simulink model "EcoSIM3_P2_C2_WIP"  (R2014b)
settings: Solver=ode1  SolverMode=SingleTasking  StartTime=0.0  StopTime=inf  FixedStep=0.01  RelTol=1e-3
PostLoadFcn:
  | %, if any(exist('dsrtsu_mdlpostloadfcn', 'file') == [2, 3, 6]), try dsrtsu_mdlpostloadfcn('Execute', bdroot); catch fprintf('Error in PostLoadFcn (dsrtsu_mdlpostloadfcn) for model "%s":\n %s\n', bdroot, lasterr); end, end,
InitFcn:
  | tic
  | %Startup_EcoSIM
values from neighbouring files (symbols this model uses):
  EngPwr = [0 5	10	15	20	25	30	35	40	45	50	55	60	65	70	75	80	85	90	95	100	105	110	115]    [Series_Maps.m]
  EngSpd = [0 477.4645 954.929 1909.858 2864.787 3819.716 4774.645 5729.574 6684.503]    [Series_Maps.m]
  EngTrq = [0	0	0	0	0	0	0	0	0	0	0	0	0	0	0	0	0	0	0	0	0	0	0	0 ... (first row only)    [Series_Maps.m]
  Power = [0 5 10 15 20 25 30]    [Series_Maps.m]
  Torque = [-50,-40,-30,-25,-20,-15,-10,-8,-6,-4,-2,0]    [Series_Maps.m]
undefined symbols (not defined in the file or in its folder): canChannel, Controls, DriveCycles, Driver, EM_EFF_MAP, EM_PwrLoss_MAP, Glbl, Overwritten_Mode, Plants, sigbuilder_block, Trialmap, Veh_Dynamics
libraries: simulink x141, canmsglib x113, fl_lib x104, canlib x89, nesl_utility x56, sdl_lib x29, dspsigops x6, dspswit3 x5, dspstat3 x2, commnoisgen2 x1, dspfdesign x1
(part 18 of 21)

== system EcoSIM3_P2_C2_WIP/Powertrain/Soft_ECUs_IO/VNT Vector/CANTx/ESS/BCM_Status ==
  ESS : Inport
  Bus Selector3 : BusSelector  OutputSignals=BCM_Status.bcm_chg_done,BCM_Status.bcm_chgc_stat,BCM_Status.bcm_cpwr_cmd,BCM_Status.bcm_cpwr_mon,BCM_Status.bcm_epo,BCM_Status.bcm_hvil_mon,BCM_Status.bcm_ibat,BCM_Status.bcm_mainc_stat,BCM_Status.bcm_on_plug,BCM_Status.bcm_ready,BCM_Status.bcm_soc,BCM_Status.bcm_vbat
  CAN Pack2 : canmsglib/CAN Pack  CANdbFile=C:\Users\EcoCAR_HIL\Documents\Khanna\EcoSIM3_P1_0_PHEV_TCU\Final_DBC\BCM_VehBus_Std.dbc  MsgList=BCM_Status  MsgName=BCM_Status  MsgIDType=Standard (11-bit identifier)  MsgIdentifier=1040  MsgLength=8  SignalInfo=bcm_alarm$14$2$2$2$1$0$1$0$0$3$#bcm_chg_done$52$1$2$2$1$0$1$0$0$1$#bcm_chgc_stat$6$2$2$2$1$0$1$0$0$2$#bcm_cool_req$53$1$2$2$1$0$1$0$0$1$#bcm_cpwr_cmd$12$1$2$2$1$0$1$0$0$1$#bcm_cpwr_mon$13$1$2$2$1$0$1$0$0$1$#bcm_epo$1$1$2$2$1$0$1$0$0$1$#bcm_gfd$16$12$2$2$1$0$2.500000e-01$0$0$1000$#bcm_hvil_mon$3$1$2$2$1$0$1$0$0$1$#bcm_ibat$40$16$2$2$1$0$2.500000e-02$-1000$-1000$500$#bcm_lls_status$54$2$2$2$1$0$1$0$0$3$#bcm_mainc_stat$4$2$2$2$1$0$1$0$0$2$#bcm_on_plug$2$1$2$2$1$0$1$0$0$1$#bcm_ready$0$1$2$2$1$0$1$0$0$1$#bcm_soc$24$8$2$2$1$0$5.000000e-01$0$0$100$#bcm_vbat$56$12$2$2$1$0$2.500000e-01$0$0$1000$#  NSignals=16  StartBits=str2num('[int32(14);int32(52);int32(6);int32(53);int32(12);int32(13);int32(1);int32(16);int32(3);int32(40);int32(54);int32(4);int32(2);int32(0);int32(24);int32(56)]')  SignalSizes=str2num('[int32(2);int32(1);int32(2);int32(1);int32(1);int32(1);int32(1);int32(12);int32(1);int32(16);int32(2);int32(2);int32(1);int32(1);int32(8);int32(12)]')  ByteOrders=str2num('[int32(2);int32(2);int32(2);int32(2);int32(2);int32(2);int32(2);int32(2);int32(2);int32(2);int32(2);int32(2);int32(2);int32(2);int32(2);int32(2)]')  DataTypes=str2num('[int32(2);int32(2);int32(2);int32(2);int32(2);int32(2);int32(2);int32(2);int32(2);int32(2);int32(2);int32(2);int32(2);int32(2);int32(2);int32(2)]')  MultiplexTypes=str2num('[int32(1);int32(1);int32(1);int32(1);int32(1);int32(1);int32(1);int32(1);int32(1);int32(1);int32(1);int32(1);int32(1);int32(1);int32(1);int32(1)]')  MultiplexValues=str2num('[double(0);double(0);double(0);double(0);double(0);double(0);double(0);double(0);double(0);double(0);double(0);double(0);double(0);double(0);double(0);double(0)]')  Factors=str2num('[double(1);double(1);double(1);double(1);double(1);double(1);double(1);double(2.500000e-01);double(1);double(2.500000e-02);double(1);double(1);double(1);double(1);double(5.000000e-01);double(2.500000e-01)]')  Offsets=str2num('[double(0);double(0);double(0);double(0);double(0);double(0);double(0);double(0);double(0);double(-1000);double(0);double(0);double(0);double(0);double(0);double(0)]')  Minimums=str2num('[double(0);double(0);double(0);double(0);double(0);double(0);double(0);double(0);double(0);double(-1000);double(0);double(0);double(0);double(0);double(0);double(0)]')  Maximums=str2num('[double(3);double(1);double(2);double(1);double(1);double(1);double(1);double(1000);double(1);double(500);double(3);double(2);double(1);double(1);double(100);double(1000)]')  Remote=off
      settings: DataFormat=CANdb specified signals
  CAN Transmit6 : canlib/CAN Transmit  BlockHandle=7345.0001  DeviceMenu=(none)  Device=Vector Virtual 1 (Channel 1)  ObjConstructor=canChannel('Vector', 'Virtual 1', 1)  EnablePeriodicTransmit=off  MessagePeriod=1.000
  Ground{2..5} (4 alike) : Ground
  Rate Transition : RateTransition
  Rate Transition1 : RateTransition
  Rate Transition10 : RateTransition  Deterministic=off
  Rate Transition11 : RateTransition  Deterministic=off
  Rate Transition9 : RateTransition  Deterministic=off
  wires:
  Rate Transition10/1 -> CAN Pack2/10
  Rate Transition9/1 -> CAN Pack2/16
  Rate Transition11/1 -> CAN Pack2/15
  Ground3/1 -> CAN Pack2/8
  Ground2/1 -> CAN Pack2/4
  Ground5/1 -> CAN Pack2/11
  Bus Selector3/3 -> CAN Pack2/5  "<bcm_cpwr_cmd>"
  Bus Selector3/4 -> CAN Pack2/6  "<bcm_cpwr_mon>"
  Bus Selector3/2 -> Rate Transition/1  "<bcm_chgc_stat>"
  ESS/1 -> Bus Selector3/1
  Bus Selector3/5 -> CAN Pack2/7  "<bcm_epo>"
  Bus Selector3/6 -> CAN Pack2/9  "<bcm_hvil_mon>"
  Bus Selector3/8 -> CAN Pack2/12  "<bcm_mainc_stat>"
  Bus Selector3/7 -> Rate Transition10/1  "<bcm_ibat>"
  Bus Selector3/9 -> CAN Pack2/13  "<bcm_on_plug>"
  Bus Selector3/10 -> CAN Pack2/14  "<bcm_ready>"
  Bus Selector3/11 -> Rate Transition11/1  "<bcm_soc>"
  Bus Selector3/12 -> Rate Transition9/1  "<bcm_vbat>"
  Rate Transition/1 -> CAN Pack2/3
  CAN Pack2/1 -> CAN Transmit6/1
  Ground4/1 -> CAN Pack2/1
  Bus Selector3/1 -> Rate Transition1/1  "<bcm_chg_done>"
  Rate Transition1/1 -> CAN Pack2/2

== system EcoSIM3_P2_C2_WIP/Powertrain/Soft_ECUs_IO/VNT Vector/CANTx/GMLAN/PPEI_Brake_Apply_Status ==
  GM : Inport
  Bus Selector3 : BusSelector  OutputSignals=PPEI_Brake_Apply_Status.BrkPdlPos
  CAN Pack1 : canmsglib/CAN Pack  CANdbFile=C:\Users\EcoCAR_HIL\Documents\Khanna\EcoSIM3_P1_0_PHEV_TCU\Final_DBC\GlobalAHS_anon GM CONFIDENTIAL.dbc  MsgList=PPEI_Brake_Apply_Status  MsgName=PPEI_Brake_Apply_Status  MsgIDType=Standard (11-bit identifier)  MsgIdentifier=241  MsgLength=6  SignalInfo=BrkAppSnsrHmPosLrnd$30$1$2$2$1$0$1$0$0$1$#BrkPdlChkData$40$17$2$2$1$0$1$0$0$131071$#BrkPdlInTrvPrt$2$2$2$2$1$0$1$0$0$3$#BrkPdlModTrvl$6$1$2$2$1$0$1$0$0$1$#BrkPdlModTrvlV$7$1$2$2$1$0$1$0$0$1$#BrkPdlPos$8$8$2$2$1$0$3.921570e-01$0$0$1.000000e+02$#BrkPdlPosGrad$16$8$2$1$1$0$40$0$-5120$5080$#BrkPedPosAlvRolngCnt$4$2$2$2$1$0$1$0$0$3$#BrkPedTrvlAchvd$1$1$2$2$1$0$1$0$0$1$#BrkPedTrvlAchvdV$0$1$2$2$1$0$1$0$0$1$#NotEventStat$28$2$2$2$1$0$1$0$0$3$#  NSignals=11  StartBits=str2num('[int32(30);int32(40);int32(2);int32(6);int32(7);int32(8);int32(16);int32(4);int32(1);int32(0);int32(28)]')  SignalSizes=str2num('[int32(1);int32(17);int32(2);int32(1);int32(1);int32(8);int32(8);int32(2);int32(1);int32(1);int32(2)]')  ByteOrders=str2num('[int32(2);int32(2);int32(2);int32(2);int32(2);int32(2);int32(2);int32(2);int32(2);int32(2);int32(2)]')  DataTypes=str2num('[int32(2);int32(2);int32(2);int32(2);int32(2);int32(2);int32(1);int32(2);int32(2);int32(2);int32(2)]')  MultiplexTypes=str2num('[int32(1);int32(1);int32(1);int32(1);int32(1);int32(1);int32(1);int32(1);int32(1);int32(1);int32(1)]')  MultiplexValues=str2num('[double(0);double(0);double(0);double(0);double(0);double(0);double(0);double(0);double(0);double(0);double(0)]')  Factors=str2num('[double(1);double(1);double(1);double(1);double(1);double(3.921570e-01);double(40);double(1);double(1);double(1);double(1)]')  Offsets=str2num('[double(0);double(0);double(0);double(0);double(0);double(0);double(0);double(0);double(0);double(0);double(0)]')  Minimums=str2num('[double(0);double(0);double(0);double(0);double(0);double(0);double(-5120);double(0);double(0);double(0);double(0)]')  Maximums=str2num('[double(1);double(131071);double(3);double(1);double(1);double(1.000000e+02);double(5080);double(3);double(1);double(1);double(3)]')  Remote=off
      settings: DataFormat=CANdb specified signals
  Ground_{1..10} (10 alike) : Ground
  Rate Transition : RateTransition
  Out1 : Outport
  wires:
  Ground_1/1 -> CAN Pack1/1
  Ground_5/1 -> CAN Pack1/5
  Ground_4/1 -> CAN Pack1/4
  Ground_6/1 -> CAN Pack1/7
  Ground_2/1 -> CAN Pack1/2
  Ground_3/1 -> CAN Pack1/3
  Ground_10/1 -> CAN Pack1/11
  Ground_7/1 -> CAN Pack1/8
  Ground_8/1 -> CAN Pack1/9
  Ground_9/1 -> CAN Pack1/10
  Bus Selector3/1 -> Rate Transition/1  "<BrkPdlPos>"
  GM/1 -> Bus Selector3/1
  Rate Transition/1 -> CAN Pack1/6
  CAN Pack1/1 -> Out1/1

== system EcoSIM3_P2_C2_WIP/Powertrain/Soft_ECUs_IO/VNT Vector/CANTx/GMLAN/PPEI_Driven_Whl_Rotational_Stat ==
  GM : Inport
  Bus Selector2 : BusSelector  OutputSignals=PPEI_Driven_Whl_Rotational_Stat.WRSLDWhlDistPlsCntr,PPEI_Driven_Whl_Rotational_Stat.WRSRDWhlDistPlsCntr
  CAN Pack4 : canmsglib/CAN Pack  CANdbFile=C:\Users\EcoCAR_HIL\Documents\Khanna\EcoSIM3_P1_0_PHEV_TCU\Final_DBC\GlobalAHS_anon GM CONFIDENTIAL.dbc  MsgList=PPEI_Driven_Whl_Rotational_Stat  MsgName=PPEI_Driven_Whl_Rotational_Stat  MsgIDType=Standard (11-bit identifier)  MsgIdentifier=193  MsgLength=8  SignalInfo=WRSLDSeqNum$4$2$2$2$1$0$1$0$0$3$#WRSLDWhlDisTpRC$6$2$2$2$1$0$1$0$0$3$#WRSLDWhlDistPlsCntr$8$10$2$2$1$0$1$0$0$1023$#WRSLDWhlDistTmstm$24$16$2$2$1$0$1$0$0$65535$#WRSLDWhlDistVal$2$1$2$2$1$0$1$0$0$1$#WRSLDWhlRotStatRst$3$1$2$2$1$0$1$0$0$1$#WRSRDSeqNum$36$2$2$2$1$0$1$0$0$3$#WRSRDWhlDisTpRC$38$2$2$2$1$0$1$0$0$3$#WRSRDWhlDistPlsCntr$40$10$2$2$1$0$1$0$0$1023$#WRSRDWhlDistTmstm$56$16$2$2$1$0$1$0$0$65535$#WRSRDWhlDistVal$34$1$2$2$1$0$1$0$0$1$#WRSRDWhlRotStatRst$35$1$2$2$1$0$1$0$0$1$#  NSignals=12  StartBits=str2num('[int32(4);int32(6);int32(8);int32(24);int32(2);int32(3);int32(36);int32(38);int32(40);int32(56);int32(34);int32(35)]')  SignalSizes=str2num('[int32(2);int32(2);int32(10);int32(16);int32(1);int32(1);int32(2);int32(2);int32(10);int32(16);int32(1);int32(1)]')  ByteOrders=str2num('[int32(2);int32(2);int32(2);int32(2);int32(2);int32(2);int32(2);int32(2);int32(2);int32(2);int32(2);int32(2)]')  DataTypes=str2num('[int32(2);int32(2);int32(2);int32(2);int32(2);int32(2);int32(2);int32(2);int32(2);int32(2);int32(2);int32(2)]')  MultiplexTypes=str2num('[int32(1);int32(1);int32(1);int32(1);int32(1);int32(1);int32(1);int32(1);int32(1);int32(1);int32(1);int32(1)]')  MultiplexValues=str2num('[double(0);double(0);double(0);double(0);double(0);double(0);double(0);double(0);double(0);double(0);double(0);double(0)]')  Factors=str2num('[double(1);double(1);double(1);double(1);double(1);double(1);double(1);double(1);double(1);double(1);double(1);double(1)]')  Offsets=str2num('[double(0);double(0);double(0);double(0);double(0);double(0);double(0);double(0);double(0);double(0);double(0);double(0)]')  Minimums=str2num('[double(0);double(0);double(0);double(0);double(0);double(0);double(0);double(0);double(0);double(0);double(0);double(0)]')  Maximums=str2num('[double(3);double(3);double(1023);double(65535);double(1);double(1);double(3);double(3);double(1023);double(65535);double(1);double(1)]')  Remote=off
      settings: DataFormat=CANdb specified signals
  CAN Transmit : canlib/CAN Transmit  BlockHandle=7430.0001  DeviceMenu=(none)  Device=Vector Virtual 1 (Channel 1)  ObjConstructor=canChannel('Vector', 'Virtual 1', 1)  EnablePeriodicTransmit=on  MessagePeriod=0.01
  Ground_{50..59} (10 alike) : Ground
  Scope1 : Scope
      settings: SaveName=ScopeData18
  Scope2 : Scope
      settings: SaveName=ScopeData23
  Out1 : Outport
  wires:
  Bus Selector2/1 -> Scope2/1, CAN Pack4/3, Scope1/1  "<WRSLDWhlDistPlsCntr>"
  Bus Selector2/2 -> CAN Pack4/9  "<WRSRDWhlDistPlsCntr>"
  Ground_57/1 -> CAN Pack4/10
  Ground_50/1 -> CAN Pack4/1
  Ground_59/1 -> CAN Pack4/12
  Ground_53/1 -> CAN Pack4/5
  Ground_52/1 -> CAN Pack4/4
  Ground_51/1 -> CAN Pack4/2
  Ground_54/1 -> CAN Pack4/6
  Ground_55/1 -> CAN Pack4/7
  Ground_56/1 -> CAN Pack4/8
  Ground_58/1 -> CAN Pack4/11
  GM/1 -> Bus Selector2/1
  CAN Pack4/1 -> CAN Transmit/1, Out1/1

== system EcoSIM3_P2_C2_WIP/Powertrain/Soft_ECUs_IO/VNT Vector/CANTx/GMLAN/PPEI_NonDrivn_Whl_Rotational_Stat ==
  GM : Inport
  Bus Selector5 : BusSelector  OutputSignals=PPEI_NonDrivn_Whl_Rotationl_Stat.WRSLNDWhlDistPCntr,PPEI_NonDrivn_Whl_Rotationl_Stat.WRSRNDWhlDistPCntr
  CAN Pack5 : canmsglib/CAN Pack  CANdbFile=C:\Users\EcoCAR_HIL\Documents\Khanna\EcoSIM3_P1_0_PHEV_TCU\Final_DBC\GlobalAHS_anon GM CONFIDENTIAL.dbc  MsgList=PPEI_NonDrivn_Whl_Rotationl_Stat  MsgName=PPEI_NonDrivn_Whl_Rotationl_Stat  MsgIDType=Standard (11-bit identifier)  MsgIdentifier=197  MsgLength=8  SignalInfo=WRSLNDSeqNum$4$2$2$2$1$0$1$0$0$3$#WRSLNDWhlDisTpRC$6$2$2$2$1$0$1$0$0$3$#WRSLNDWhlDistPCntr$8$10$2$2$1$0$1$0$0$1023$#WRSLNDWhlDistTstm$24$16$2$2$1$0$1$0$0$65535$#WRSLNDWhlDistVal$2$1$2$2$1$0$1$0$0$1$#WRSLNDWhlRotStRst$3$1$2$2$1$0$1$0$0$1$#WRSRNDSeqNum$36$2$2$2$1$0$1$0$0$3$#WRSRNDWhlDisTpRC$38$2$2$2$1$0$1$0$0$3$#WRSRNDWhlDistPCntr$40$10$2$2$1$0$1$0$0$1023$#WRSRNDWhlDistTstm$56$16$2$2$1$0$1$0$0$65535$#WRSRNDWhlDistVal$34$1$2$2$1$0$1$0$0$1$#WRSRNDWhlRotStRst$35$1$2$2$1$0$1$0$0$1$#  NSignals=12  StartBits=str2num('[int32(4);int32(6);int32(8);int32(24);int32(2);int32(3);int32(36);int32(38);int32(40);int32(56);int32(34);int32(35)]')  SignalSizes=str2num('[int32(2);int32(2);int32(10);int32(16);int32(1);int32(1);int32(2);int32(2);int32(10);int32(16);int32(1);int32(1)]')  ByteOrders=str2num('[int32(2);int32(2);int32(2);int32(2);int32(2);int32(2);int32(2);int32(2);int32(2);int32(2);int32(2);int32(2)]')  DataTypes=str2num('[int32(2);int32(2);int32(2);int32(2);int32(2);int32(2);int32(2);int32(2);int32(2);int32(2);int32(2);int32(2)]')  MultiplexTypes=str2num('[int32(1);int32(1);int32(1);int32(1);int32(1);int32(1);int32(1);int32(1);int32(1);int32(1);int32(1);int32(1)]')  MultiplexValues=str2num('[double(0);double(0);double(0);double(0);double(0);double(0);double(0);double(0);double(0);double(0);double(0);double(0)]')  Factors=str2num('[double(1);double(1);double(1);double(1);double(1);double(1);double(1);double(1);double(1);double(1);double(1);double(1)]')  Offsets=str2num('[double(0);double(0);double(0);double(0);double(0);double(0);double(0);double(0);double(0);double(0);double(0);double(0)]')  Minimums=str2num('[double(0);double(0);double(0);double(0);double(0);double(0);double(0);double(0);double(0);double(0);double(0);double(0)]')  Maximums=str2num('[double(3);double(3);double(1023);double(65535);double(1);double(1);double(3);double(3);double(1023);double(65535);double(1);double(1)]')  Remote=off
      settings: DataFormat=CANdb specified signals
  CAN Transmit : canlib/CAN Transmit  BlockHandle=7468.0001  DeviceMenu=(none)  Device=Vector Virtual 1 (Channel 1)  ObjConstructor=canChannel('Vector', 'Virtual 1', 1)  EnablePeriodicTransmit=on  MessagePeriod=0.01
  Ground_{60..69} (10 alike) : Ground
  Out1 : Outport
  wires:
  Bus Selector5/2 -> CAN Pack5/9  "<WRSRNDWhlDistPCntr>"
  Bus Selector5/1 -> CAN Pack5/3  "<WRSLNDWhlDistPCntr>"
  Ground_60/1 -> CAN Pack5/1
  Ground_69/1 -> CAN Pack5/12
  Ground_63/1 -> CAN Pack5/5
  Ground_61/1 -> CAN Pack5/2
  Ground_66/1 -> CAN Pack5/8
  Ground_67/1 -> CAN Pack5/10
  Ground_68/1 -> CAN Pack5/11
  Ground_65/1 -> CAN Pack5/7
  Ground_62/1 -> CAN Pack5/4
  GM/1 -> Bus Selector5/1
  CAN Pack5/1 -> CAN Transmit/1, Out1/1
  Ground_64/1 -> CAN Pack5/6

== system EcoSIM3_P2_C2_WIP/Powertrain/Soft_ECUs_IO/VNT Vector/CANTx/GMLAN/PPEI_Platform_General_Status ==
  GM : Inport
  Bus Selector1 : BusSelector  OutputSignals=PPEI_Platform_General_Status.SysPwrMd
  CAN Pack2 : canmsglib/CAN Pack  CANdbFile=C:\Users\EcoCAR_HIL\Documents\Khanna\EcoSIM3_P1_0_PHEV_TCU\Final_DBC\GlobalAHS_anon GM CONFIDENTIAL.dbc  MsgList=PPEI_Platform_General_Status  MsgName=PPEI_Platform_General_Status  MsgIDType=Standard (11-bit identifier)  MsgIdentifier=497  MsgLength=8  SignalInfo=ACCmpsrFldOn$63$1$2$2$1$0$1$0$0$1$#ACCompModReq$11$2$2$2$1$0$1$0$0$3$#ACCompNormLd$48$8$2$2$1$0$1.000000e-01$0$0$2.550000e+01$#ACCompNormLdV$10$1$2$2$1$0$1$0$0$1$#ACCompSysVDA$9$1$2$2$1$0$1$0$0$1$#ACCompSysVDM$60$1$2$2$1$0$1$0$0$1$#AirbgVDA$57$1$2$2$1$0$1$0$0$1$#BkupPwrModeMstrVDA$7$1$2$2$1$0$1$0$0$1$#BkupPwrModeMstrVDM$61$1$2$2$1$0$1$0$0$1$#DispMeasSys$59$1$2$2$1$0$1$0$0$1$#ElvtdIdlCstStReq$32$2$2$2$1$0$1$0$0$3$#EngOilLfRstRq$37$1$2$2$1$0$1$0$0$1$#FuelFltLfRstRqd$56$1$2$2$1$0$1$0$0$1$#ImmblzrPreRelPswdStat$8$1$2$2$1$0$1$0$0$1$#ImmblzrPreRelPswrd$24$16$2$2$1$0$1$0$0$65535$#PMMAccTrmSt$2$1$2$2$1$0$1$0$0$1$#PMMRunCrkTrmSt$3$1$2$2$1$0$1$0$0$1$#PTORSMstrEngShtReq$13$1$2$2$1$0$1$0$0$1$#PTORmStMsEngStRq$14$1$2$2$1$0$1$0$0$1$#PrkBrkSwAtv$36$1$2$2$1$0$1$0$0$1$#PrkBrkVDA$35$1$2$2$1$0$1$0$0$1$#PrkBrkVDM$62$1$2$2$1$0$1$0$0$1$#RmVehStrRq$15$1$2$2$1$0$1$0$0$1$#SIRDpl$58$1$2$2$1$0$1$0$0$1$#SysBkUpPwrMd$4$2$2$2$1$0$1$0$0$3$#SysBkupPwrMdEn$6$1$2$2$1$0$1$0$0$1$#SysPwrMd$0$2$2$2$1$0$1$0$0$3$#ThrtlPrgrsnReq$38$2$2$2$1$0$1$0$0$3$#TrStLgMdAtv$34$1$2$2$1$0$1$0$0$1$#  NSignals=29  StartBits=str2num('[int32(63);int32(11);int32(48);int32(10);int32(9);int32(60);int32(57);int32(7);int32(61);int32(59);int32(32);int32(37);int32(56);int32(8);int32(24);int32(2);int32(3);int32(13);int32(14);int32(36);int32(35);int32(62);int32(15);int32(58);int32(4);int32(6);int32(0);int32(38);int32(34)]')  SignalSizes=str2num('[int32(1);int32(2);int32(8);int32(1);int32(1);int32(1);int32(1);int32(1);int32(1);int32(1);int32(2);int32(1);int32(1);int32(1);int32(16);int32(1);int32(1);int32(1);int32(1);int32(1);int32(1);int32(1);int32(1);int32(1);int32(2);int32(1);int32(2);int32(2);int32(1)]')  ByteOrders=str2num('[int32(2);int32(2);int32(2);int32(2);int32(2);int32(2);int32(2);int32(2);int32(2);int32(2);int32(2);int32(2);int32(2);int32(2);int32(2);int32(2);int32(2);int32(2);int32(2);int32(2);int32(2);int32(2);int32(2);int32(2);int32(2);int32(2);int32(2);int32(2);int32(2)]')  DataTypes=str2num('[int32(2);int32(2);int32(2);int32(2);int32(2);int32(2);int32(2);int32(2);int32(2);int32(2);int32(2);int32(2);int32(2);int32(2);int32(2);int32(2);int32(2);int32(2);int32(2);int32(2);int32(2);int32(2);int32(2);int32(2);int32(2);int32(2);int32(2);int32(2);int32(2)]')  MultiplexTypes=str2num('[int32(1);int32(1);int32(1);int32(1);int32(1);int32(1);int32(1);int32(1);int32(1);int32(1);int32(1);int32(1);int32(1);int32(1);int32(1);int32(1);int32(1);int32(1);int32(1);int32(1);int32(1);int32(1);int32(1);int32(1);int32(1);int32(1);int32(1);int32(1);int32(1)]')  MultiplexValues=str2num('[double(0);double(0);double(0);double(0);double(0);double(0);double(0);double(0);double(0);double(0);double(0);double(0);double(0);double(0);double(0);double(0);double(0);double(0);double(0);double(0);double(0);double(0);double(0);double(0);double(0);double(0);double(0);double(0);double(0)]')  Factors=str2num('[double(1);double(1);double(1.000000e-01);double(1);double(1);double(1);double(1);double(1);double(1);double(1);double(1);double(1);double(1);double(1);double(1);double(1);double(1);double(1);double(1);double(1);double(1);double(1);double(1);double(1);double(1);double(1);double(1);double(1);double(1)]')  Offsets=str2num('[double(0);double(0);double(0);double(0);double(0);double(0);double(0);double(0);double(0);double(0);double(0);double(0);double(0);double(0);double(0);double(0);double(0);double(0);double(0);double(0);double(0);double(0);double(0);double(0);double(0);double(0);double(0);double(0);double(0)]')  Minimums=str2num('[double(0);double(0);double(0);double(0);double(0);double(0);double(0);double(0);double(0);double(0);double(0);double(0);double(0);double(0);double(0);double(0);double(0);double(0);double(0);double(0);double(0);double(0);double(0);double(0);double(0);double(0);double(0);double(0);double(0)]')  Maximums=str2num('[double(1);double(3);double(2.550000e+01);double(1);double(1);double(1);double(1);double(1);double(1);double(1);double(3);double(1);double(1);double(1);double(65535);double(1);double(1);double(1);double(1);double(1);double(1);double(1);double(1);double(1);double(3);double(1);double(3);double(3);double(1)]')  Remote=off
      settings: DataFormat=CANdb specified signals
  Ground_{11..38} (28 alike) : Ground
  Rate Transition : RateTransition
  Out1 : Outport
  wires:
  Ground_29/1 -> CAN Pack2/19
  CAN Pack2/1 -> Out1/1
  Ground_32/1 -> CAN Pack2/22
  Ground_35/1 -> CAN Pack2/25
  Ground_11/1 -> CAN Pack2/1
  Ground_27/1 -> CAN Pack2/17
  Ground_15/1 -> CAN Pack2/5
  Ground_37/1 -> CAN Pack2/28
  Ground_13/1 -> CAN Pack2/3
  Ground_16/1 -> CAN Pack2/6
  Ground_24/1 -> CAN Pack2/14
  Ground_25/1 -> CAN Pack2/15
  Ground_14/1 -> CAN Pack2/4
  Ground_28/1 -> CAN Pack2/18
  Ground_31/1 -> CAN Pack2/21
  Ground_38/1 -> CAN Pack2/29
  Ground_21/1 -> CAN Pack2/11
  Ground_26/1 -> CAN Pack2/16
  Ground_30/1 -> CAN Pack2/20
  Ground_20/1 -> CAN Pack2/10
  Ground_17/1 -> CAN Pack2/7
  Ground_22/1 -> CAN Pack2/12
  Ground_36/1 -> CAN Pack2/26
  Ground_33/1 -> CAN Pack2/23
  Ground_18/1 -> CAN Pack2/8
  Ground_34/1 -> CAN Pack2/24
  Ground_12/1 -> CAN Pack2/2
  Ground_19/1 -> CAN Pack2/9
  Ground_23/1 -> CAN Pack2/13
  Bus Selector1/1 -> Rate Transition/1  "<SysPwrMd>"
  GM/1 -> Bus Selector1/1
  Rate Transition/1 -> CAN Pack2/27

== system EcoSIM3_P2_C2_WIP/Powertrain/Soft_ECUs_IO/VNT Vector/CANTx/GMLAN/PPEI_Vehicle_Speed_and_Distance ==
  GM : Inport
  Bus Selector4 : BusSelector  OutputSignals=PPEI_Vehicle_Speed_and_Distance.VehSpdAvgDrvn
  CAN Pack3 : canmsglib/CAN Pack  CANdbFile=C:\Users\EcoCAR_HIL\Documents\Khanna\EcoSIM3_P1_0_PHEV_TCU\Final_DBC\GlobalAHS_anon GM CONFIDENTIAL.dbc  MsgList=PPEI_Vehicle_Speed_and_Distance  MsgName=PPEI_Vehicle_Speed_and_Distance  MsgIDType=Standard (11-bit identifier)  MsgIdentifier=1001  MsgLength=8  SignalInfo=DistRollCntAvgDrvn$24$13$2$2$1$0$1.250000e-01$0$0$1.023875e+03$#DistRollCntAvgDrvnSrc$55$1$2$2$1$0$1$0$0$1$#DistRollCntAvgDrvnV$22$1$2$2$1$0$1$0$0$1$#DstRolCntAvNDrRstOc$53$1$2$2$1$0$1$0$0$1$#DstRolCntAvgDrnRstOc$21$1$2$2$1$0$1$0$0$1$#DstRolCntAvgNonDrvn$56$13$2$2$1$0$1.250000e-01$0$0$1.023875e+03$#DstRolCntAvgNonDrvnV$54$1$2$2$1$0$1$0$0$1$#VehSpdAvgDrvn$8$15$2$2$1$0$1.562500e-02$0$0$5.119844e+02$#VehSpdAvgDrvnSrc$23$1$2$2$1$0$1$0$0$1$#VehSpdAvgDrvnV$7$1$2$2$1$0$1$0$0$1$#VehSpdAvgNDrvn$40$15$2$2$1$0$1.562500e-02$0$0$5.119844e+02$#VehSpdAvgNDrvnV$39$1$2$2$1$0$1$0$0$1$#  NSignals=12  StartBits=str2num('[int32(24);int32(55);int32(22);int32(53);int32(21);int32(56);int32(54);int32(8);int32(23);int32(7);int32(40);int32(39)]')  SignalSizes=str2num('[int32(13);int32(1);int32(1);int32(1);int32(1);int32(13);int32(1);int32(15);int32(1);int32(1);int32(15);int32(1)]')  ByteOrders=str2num('[int32(2);int32(2);int32(2);int32(2);int32(2);int32(2);int32(2);int32(2);int32(2);int32(2);int32(2);int32(2)]')  DataTypes=str2num('[int32(2);int32(2);int32(2);int32(2);int32(2);int32(2);int32(2);int32(2);int32(2);int32(2);int32(2);int32(2)]')  MultiplexTypes=str2num('[int32(1);int32(1);int32(1);int32(1);int32(1);int32(1);int32(1);int32(1);int32(1);int32(1);int32(1);int32(1)]')  MultiplexValues=str2num('[double(0);double(0);double(0);double(0);double(0);double(0);double(0);double(0);double(0);double(0);double(0);double(0)]')  Factors=str2num('[double(1.250000e-01);double(1);double(1);double(1);double(1);double(1.250000e-01);double(1);double(1.562500e-02);double(1);double(1);double(1.562500e-02);double(1)]')  Offsets=str2num('[double(0);double(0);double(0);double(0);double(0);double(0);double(0);double(0);double(0);double(0);double(0);double(0)]')  Minimums=str2num('[double(0);double(0);double(0);double(0);double(0);double(0);double(0);double(0);double(0);double(0);double(0);double(0)]')  Maximums=str2num('[double(1.023875e+03);double(1);double(1);double(1);double(1);double(1.023875e+03);double(1);double(5.119844e+02);double(1);double(1);double(5.119844e+02);double(1)]')  Remote=off
      settings: DataFormat=CANdb specified signals
  Ground_{39..49} (11 alike) : Ground
  Rate Transition : RateTransition
  Out1 : Outport
  wires:
  CAN Pack3/1 -> Out1/1
  Ground_47/1 -> CAN Pack3/10
  Ground_45/1 -> CAN Pack3/7
  Ground_44/1 -> CAN Pack3/6
  Ground_46/1 -> CAN Pack3/9
  Ground_49/1 -> CAN Pack3/12
  Ground_48/1 -> CAN Pack3/11
  Ground_42/1 -> CAN Pack3/4
  Ground_40/1 -> CAN Pack3/2
  Ground_39/1 -> CAN Pack3/1
  Ground_43/1 -> CAN Pack3/5
  Ground_41/1 -> CAN Pack3/3
  Bus Selector4/1 -> Rate Transition/1  "<VehSpdAvgDrvn>"
  GM/1 -> Bus Selector4/1
  Rate Transition/1 -> CAN Pack3/8

== system EcoSIM3_P2_C2_WIP/Supervisory Controller/Functional Safety1/Functional Safety Algorithm/Fault Detection (Team Developed)/Torque Security Faults/Torque Comparisons ==
  Torque Estimates : Inport
  Torque Feedbacks : Inport  Port=2
  Torque Requests : Inport  Port=3
  BAS Torque Comparison : Subsystem  Commented=on
  Belt Coupler Torque Comparison : Subsystem  Commented=on
  Bus Creator : BusCreator  Inputs=3
  Bus Creator1 : BusCreator  Inputs=9
  Clutch Torque Comparison : Subsystem  Commented=on
  Electric Motor Torque Comparison : Subsystem
  Engine Torque Comparison : Subsystem  Commented=on
  PTU Torque Comparison : Subsystem  Commented=on
  Rear Diff Torque Comparison : Subsystem  Commented=on
  Trans Torque Comparison : Subsystem  Commented=on
  Wheel Torque Comparison : Subsystem  Commented=on
  Faults : Outport
  wires:
  Bus Creator1/1 -> Faults/1  "Trq_Security_Faults"
  Torque Requests/1 -> Bus Creator/3
  Torque Feedbacks/1 -> Bus Creator/2
  Torque Estimates/1 -> Bus Creator/1
  Clutch Torque Comparison/1(Out1) -> Bus Creator1/9
  Rear Diff Torque Comparison/1(Out1) -> Bus Creator1/8
  PTU Torque Comparison/1(Out1) -> Bus Creator1/7
  Belt Coupler Torque Comparison/1(Out1) -> Bus Creator1/6
  Trans Torque Comparison/1(Out1) -> Bus Creator1/5
  Electric Motor Torque Comparison/1(Out1) -> Bus Creator1/4
  BAS Torque Comparison/1(Out1) -> Bus Creator1/3
  Wheel Torque Comparison/1(Out1) -> Bus Creator1/1
  Bus Creator/1 -> Wheel Torque Comparison/1(In1), Engine Torque Comparison/1(In1), BAS Torque Comparison/1(In1), Electric Motor Torque Comparison/1(In1), Belt Coupler Torque Comparison/1(In1), PTU Torque Comparison/1(In1), Rear Diff Torque Comparison/1(In1), Clutch Torque Comparison/1(In1), Trans Torque Comparison/1(In1)
  Engine Torque Comparison/1(Out1) -> Bus Creator1/2

== system EcoSIM3_P2_C2_WIP/Supervisory Controller/Functional Safety1/Functional Safety Algorithm/Fault Detection (Team Developed)/Torque Security Faults/Torque Estimation ==
  Veh Mass Est : Inport
  ECU/Sensor Signals : Inport  Port=2
  BAS Torque Estimation : Subsystem  Commented=on
  Belt Coupler Torque Estimation : Subsystem  Commented=on
  Bus Creator : BusCreator  Inputs=9
  Clutch Torque Estimation : Subsystem  Commented=on
  Electric Motor Torque Estimation : Subsystem
  Engine Torque Estimation : Subsystem  Commented=on
  PTU Torque Estimation : Subsystem  Commented=on
  Rear Diff Torque Estimation : Subsystem  Commented=on
  Trans Torque Estimation : Subsystem  Commented=on
  Wheel Torque Estimation : Subsystem  Commented=on
  Torque_Estimates : Outport
  wires:
  Bus Creator/1 -> Torque_Estimates/1  "Torque_Estimates"
  Clutch Torque Estimation/1(Out1) -> Bus Creator/9
  Rear Diff Torque Estimation/1(Out1) -> Bus Creator/8
  PTU Torque Estimation/1(Out1) -> Bus Creator/7
  Belt Coupler Torque Estimation/1(Out1) -> Bus Creator/6
  Trans Torque Estimation/1(Out1) -> Bus Creator/5
  Electric Motor Torque Estimation/1(Out1) -> Bus Creator/4
  BAS Torque Estimation/1(Out1) -> Bus Creator/3
  Wheel Torque Estimation/1(Whl Trq Est) -> Bus Creator/1
  ECU/Sensor Signals/1 -> Wheel Torque Estimation/2(ECU/Sensor Signals), Engine Torque Estimation/1(In1), BAS Torque Estimation/1(In1), Electric Motor Torque Estimation/1(In1), Trans Torque Estimation/1(In1), Belt Coupler Torque Estimation/1(In1), PTU Torque Estimation/1(In1), Rear Diff Torque Estimation/1(In1), Clutch Torque Estimation/1(In1)
  Veh Mass Est/1 -> Wheel Torque Estimation/1(Veh Mass Est)
  Engine Torque Estimation/1(Out1) -> Bus Creator/2

== system EcoSIM3_P2_C2_WIP/Supervisory Controller/Functional Safety1/Functional Safety Algorithm/Fault Detection (Team Developed)/Torque Security Faults/Vehicle Mass Estimation ==
  In1 : Inport
  Add : Sum  Inputs=+++-
  Belt Coupler : Subsystem
  Bus Selector : BusSelector  OutputSignals=EM_Transmit.EM_Torque_Out_Nm,Trans_Transmit.Actual_Gear,ICE_Transmit.ICE_Torque_Cmd_Nm,BAS_Transmit.BAS_Torque_Command_Nm,Vehicle_Speed_meter_per_s
  Constant : Constant  Value=0
  Constant1 : Constant  Value=2000
  Derivative : Derivative
  Driveline : Subsystem
  Driveline1 : Subsystem
  Driveline2 : Subsystem
  Ground : Ground
  Lowpass Filter : dspfdesign/Lowpass Filter
  Memory1 : Memory  X0=2000  InheritSampleTime=on
  Product : Product  Inputs=*/
  Resistance Forces : Subsystem
  Scope : Scope
      settings: YMin=-28387834003.67816  YMax=8492617632.78235
  Scope1 : Scope
      settings: YMin=-10  YMax=10  SaveName=ScopeData2
  Scope5 : Scope
      settings: YMin=76.14688  YMax=848.53208  SaveName=ScopeData6
  Terminator : Terminator
  Terminator1 : Terminator
  Trans : Subsystem
  Trans1 : Subsystem
  Transfer Fcn : TransferFcn  Denominator=[1 1]
  Veh Mass Est : Outport
  wires:
  Constant1/1 -> Resistance Forces/3(Vehicle_Mass [kg])
  Ground/1 -> Veh Mass Est/1
  Memory1/1 -> Terminator1/1
  Bus Selector/5 -> Resistance Forces/1(Vehicle_Speed [m/s]), Derivative/1  "<Vehicle_Speed_meter_per_s>"
  Bus Selector/4 -> Belt Coupler/1(BAS Torque)  "<BAS_Torque_Command_Nm>"
  Bus Selector/3 -> Trans/2(ICE_Torque)  "<ICE_Torque_Cmd_Nm>"
  Bus Selector/2 -> Trans/1(Current Gear), Trans1/1(Current Gear)  "<Actual_Gear>"
  Bus Selector/1 -> Driveline/1(EM_Torque)  "<EM_Torque_Out_Nm>"
  Constant/1 -> Resistance Forces/2(Grade [%])
  Transfer Fcn/1 -> Memory1/1, Terminator/1, Scope1/1  "Veh_Mass_Est_kg"
  Resistance Forces/1(Road_Load_Force [N]) -> Add/4, Scope5/1
  Trans1/1(Out1) -> Driveline2/1(In1)
  Belt Coupler/1(Out1) -> Trans1/2(In1)
  Trans/1(Out1) -> Driveline1/1(In1)
  Driveline2/1(Out1) -> Add/3  "BAS_Force_N"
  Driveline1/1(Out1) -> Add/2  "ICE_Force_N"
  Driveline/1(Out1) -> Add/1  "EM_Force_N"
  In1/1 -> Bus Selector/1
  Derivative/1 -> Product/2  "Veh_accel_m_s2"
  Add/1 -> Product/1  "Total_Trac_Force_N"
  Product/1 -> Scope/1, Transfer Fcn/1

== system EcoSIM3_P2_C2_WIP/Supervisory Controller/Mode Operation/Engine Only /Subsystem/Engine Torque Calc/Max Torque Calculation ==
  In1 : Inport
  Gear : Inport  Port=2
  Calibration Factor : Gain
  Divide2 : Product  Inputs=**
  Max Torque : Lookup_n-D  NumberOfTableDimensions=1  BreakpointsForDimension1=Plants.ICE.Mdl.Plant.Max_Trq.w  Table=Plants.ICE.Mdl.Plant.Max_Trq.Trq  InternalRulePriority=Speed  RndMeth=Simplest  InputSameDT=on
  RearGR3 : Gain  Gain=2.77
  TRAN GR2 : Lookup_n-D  NumberOfTableDimensions=1  BreakpointsForDimension1=[1,2,3,4,5]  Table=Plants.Trans.Mdl.Plant.GR  ExtrapMethod=Clip  InternalRulePriority=Speed  RndMeth=Simplest  InputSameDT=on
  "Engine Torque " : Outport
  wires:
  RearGR3/1 -> Divide2/1
  Calibration Factor/1 -> RearGR3/1
  Max Torque/1 -> Calibration Factor/1  "Engine Torque"
  Divide2/1 -> "Engine Torque "/1
  In1/1 -> Max Torque/1
  Gear/1 -> TRAN GR2/1
  TRAN GR2/1 -> Divide2/2

== system EcoSIM3_P2_C2_WIP/Supervisory Controller/Mode Operation/Engine Only /Subsystem/Engine Torque Calc/Speed Calculations ==
  "Vehicle Speed m/s " : Inport
  Gear Current : Inport  Port=2
  Gain1 : Gain  Gain=2/Plants.Rear_wh.tire_diameter
  Gain2 : Gain  Gain=2.77
  Product : Product
  TRAN GR : Lookup_n-D  NumberOfTableDimensions=1  BreakpointsForDimension1=[1,2,3,4,5]  Table=Plants.Trans.Mdl.Plant.GR  ExtrapMethod=Clip  InternalRulePriority=Speed  RndMeth=Simplest  InputSameDT=on
  Engine Speed : Outport
  wires:
  "Vehicle Speed m/s "/1 -> Gain1/1
  Gain2/1 -> Product/2
  Gain1/1 -> Gain2/1
  Product/1 -> Engine Speed/1
  Gear Current/1 -> TRAN GR/1
  TRAN GR/1 -> Product/1

== system EcoSIM3_P2_C2_WIP/Supervisory Controller/Mode Operation/Engine Start /BAS_Signals1/Subsystem/Delay ==
  BAS_Speed_Rad_per_sec : Inport
  Memory : Memory
  Transfer Fcn1 : TransferFcn  Denominator=[1 1]
  Transport Delay : TransportDelay  Commented=on  DelayTime=0
  Pre_BAS_Speed_Rad_per_sec : Outport
  wires:
  Memory/1 -> Pre_BAS_Speed_Rad_per_sec/1
  BAS_Speed_Rad_per_sec/1 -> Memory/1

== system EcoSIM3_P2_C2_WIP/Supervisory Controller/Mode Operation/Series1/BAS_Signals/Enabled Subsystem1/Delay ==
  BAS_Speed_Rad_per_sec : Inport
  Memory : Memory
  Transfer Fcn1 : TransferFcn  Denominator=[1 1]
  Transport Delay : TransportDelay  Commented=on  DelayTime=0
  Pre_BAS_Speed_Rad_per_sec : Outport
  wires:
  Memory/1 -> Pre_BAS_Speed_Rad_per_sec/1
  BAS_Speed_Rad_per_sec/1 -> Memory/1

== system EcoSIM3_P2_C2_WIP/Supervisory Controller/Supervisory_IO/VNT Vector/CAN Tx/BAS/SetLimits ==
  In1 : Inport
  Bus Selector1 : BusSelector  OutputSignals=BAS_Infineon_Messages.Code,BAS_Infineon_Messages.ID_Limit,BAS_Infineon_Messages.IQ_Limit,BAS_Infineon_Messages.Write
  CAN Pack1 : canmsglib/CAN Pack  CANdbFile=C:\Box Sync\EcoCAR 3\SMS\EcoSIM3_P2_C2\MIL\Final_DBC\InfineonInverter.dbc  MsgList=SetLimits  MsgName=SetLimits  MsgIDType=Standard (11-bit identifier)  MsgIdentifier=272  MsgLength=8  SignalInfo=Checksum2$0$8$1$2$1$0$1$0$0$255$#Code$16$8$1$2$2$0$1$0$0$2$#Counter2$8$4$1$2$1$0$1$0$0$15$#ID_Limit$48$16$1$1$3$1$3.125000e-02$0$-1024$1.023969e+03$#IQ_Limit$32$16$1$1$3$1$3.125000e-02$0$-1024$1.023969e+03$#Reserved2$12$2$1$2$1$0$1$0$0$3$#Reserved3$15$1$1$2$1$0$1$0$0$1$#Write$14$1$1$2$1$0$1$0$0$1$#  NSignals=8  StartBits=str2num('[int32(0);int32(16);int32(8);int32(48);int32(32);int32(12);int32(15);int32(14)]')  SignalSizes=str2num('[int32(8);int32(8);int32(4);int32(16);int32(16);int32(2);int32(1);int32(1)]')  ByteOrders=str2num('[int32(1);int32(1);int32(1);int32(1);int32(1);int32(1);int32(1);int32(1)]')  DataTypes=str2num('[int32(2);int32(2);int32(2);int32(1);int32(1);int32(2);int32(2);int32(2)]')  MultiplexTypes=str2num('[int32(1);int32(2);int32(1);int32(3);int32(3);int32(1);int32(1);int32(1)]')  MultiplexValues=str2num('[double(0);double(0);double(0);double(1);double(1);double(0);double(0);double(0)]')  Factors=str2num('[double(1);double(1);double(1);double(3.125000e-02);double(3.125000e-02);double(1);double(1);double(1)]')  Offsets=str2num('[double(0);double(0);double(0);double(0);double(0);double(0);double(0);double(0)]')  Minimums=str2num('[double(0);double(0);double(0);double(-1024);double(-1024);double(0);double(0);double(0)]')  Maximums=str2num('[double(255);double(2);double(15);double(1.023969e+03);double(1.023969e+03);double(3);double(1);double(1)]')  Remote=off
      settings: DataFormat=CANdb specified signals
  Ground_{1..4} (4 alike) : Ground
  Rate Transition{1..4} (4 alike) : RateTransition
  Out1 : Outport
  wires:
  CAN Pack1/1 -> Out1/1
  Ground_1/1 -> CAN Pack1/1
  Ground_2/1 -> CAN Pack1/3
  Ground_3/1 -> CAN Pack1/6
  Ground_4/1 -> CAN Pack1/7
  Bus Selector1/4 -> Rate Transition4/1  "<Write>"
  Bus Selector1/3 -> Rate Transition2/1  "<IQ_Limit>"
  Bus Selector1/2 -> Rate Transition1/1  "<ID_Limit>"
  Bus Selector1/1 -> Rate Transition3/1  "<Code>"
  In1/1 -> Bus Selector1/1
  Rate Transition3/1 -> CAN Pack1/2
  Rate Transition1/1 -> CAN Pack1/4
  Rate Transition2/1 -> CAN Pack1/5
  Rate Transition4/1 -> CAN Pack1/8

== system EcoSIM3_P2_C2_WIP/Supervisory Controller/Supervisory_IO/VNT Vector/CAN Tx/BAS/SetValues ==
  In1 : Inport
  Bus Selector2 : BusSelector  OutputSignals=BAS_Infineon_Messages.ID_Command,BAS_Infineon_Messages.IQ_Command,BAS_Infineon_Messages.ModeReq
  CAN Pack2 : canmsglib/CAN Pack  CANdbFile=C:\Box Sync\EcoCAR 3\SMS\EcoSIM3_P2_C2\MIL\Final_DBC\InfineonInverter.dbc  MsgList=SetValues  MsgName=SetValues  MsgIDType=Standard (11-bit identifier)  MsgIdentifier=256  MsgLength=8  SignalInfo=Checksum1$0$8$1$2$1$0$1$0$-Inf$Inf$#Counter1$8$8$1$2$1$0$1$0$0$15$#ID_Command$32$16$1$1$3$1$3.125000e-02$0$-1024$1.023969e+03$#IQ_Command$16$16$1$1$3$1$3.125000e-02$0$-1024$1.023969e+03$#ModeReq$48$8$1$2$2$0$1$0$0$2$#Reserved1$56$8$1$2$1$0$1$0$0$255$#Speed_Command$16$16$1$1$3$2$5.000000e-01$0$-16384$1.638350e+04$#  NSignals=7  StartBits=str2num('[int32(0);int32(8);int32(32);int32(16);int32(48);int32(56);int32(16)]')  SignalSizes=str2num('[int32(8);int32(8);int32(16);int32(16);int32(8);int32(8);int32(16)]')  ByteOrders=str2num('[int32(1);int32(1);int32(1);int32(1);int32(1);int32(1);int32(1)]')  DataTypes=str2num('[int32(2);int32(2);int32(1);int32(1);int32(2);int32(2);int32(1)]')  MultiplexTypes=str2num('[int32(1);int32(1);int32(3);int32(3);int32(2);int32(1);int32(3)]')  MultiplexValues=str2num('[double(0);double(0);double(1);double(1);double(0);double(0);double(2)]')  Factors=str2num('[double(1);double(1);double(3.125000e-02);double(3.125000e-02);double(1);double(1);double(5.000000e-01)]')  Offsets=str2num('[double(0);double(0);double(0);double(0);double(0);double(0);double(0)]')  Minimums=str2num('[double(-Inf);double(0);double(-1024);double(-1024);double(0);double(0);double(-16384)]')  Maximums=str2num('[double(Inf);double(15);double(1.023969e+03);double(1.023969e+03);double(2);double(255);double(1.638350e+04)]')  Remote=off
      settings: DataFormat=CANdb specified signals
  Ground_{5..8} (4 alike) : Ground
  Rate Transition1 : RateTransition
  Rate Transition2 : RateTransition
  Rate Transition4 : RateTransition
  Out1 : Outport
  wires:
  Ground_6/1 -> CAN Pack2/2
  Ground_8/1 -> CAN Pack2/7
  Ground_7/1 -> CAN Pack2/6
  CAN Pack2/1 -> Out1/1
  Ground_5/1 -> CAN Pack2/1
  Bus Selector2/3 -> Rate Transition2/1  "<ModeReq>"
  Bus Selector2/2 -> Rate Transition1/1  "<IQ_Command>"
  In1/1 -> Bus Selector2/1
  Bus Selector2/1 -> Rate Transition4/1  "<ID_Command>"
  Rate Transition4/1 -> CAN Pack2/3
  Rate Transition2/1 -> CAN Pack2/5
  Rate Transition1/1 -> CAN Pack2/4

== system EcoSIM3_P2_C2_WIP/Powertrain/Electric Motor /Soft ECU/Algorithm/Startup_Shutdown/Temperature Values Dummy/ESS_Over_Temp_Fault ==
  In1 : Inport
  Bus Selector1 : BusSelector  OutputSignals=Temp_deg_C,EM_Inverter_OverTemp_Trigger
  Switch : Switch  Criteria=u2 > Threshold  Threshold=0.5
  Out1 : Outport
  wires:
  In1/1 -> Switch/3
  Switch/1 -> Out1/1
  Bus Selector1/2 -> Switch/2  "<EM_Inverter_OverTemp_Trigger>"
  [EM_Inverter_Over_temperature_Trigger] -> Bus Selector1/1
  Bus Selector1/1 -> Switch/1  "<Temp_deg_C>"

== system EcoSIM3_P2_C2_WIP/Powertrain/Electrical Storage System/ ESS Model/Plant/Electrical Plant Model/OCV Estimation/Charge ==
  SOC [%] : Inport
  1-D Lookup Table1 : Lookup_n-D  NumberOfTableDimensions=1  BreakpointsForDimension1=Plants.ESS.Mdl.Plant.EPM.OCV_Est.SOC  Table=Plants.ESS.Mdl.Plant.EPM.OCV_Est.OCV_Charge  InternalRulePriority=Speed  RndMeth=Simplest  InputSameDT=on
  OCV [V] : Outport
  wires:
  SOC [%]/1 -> 1-D Lookup Table1/1
  1-D Lookup Table1/1 -> OCV [V]/1

== system EcoSIM3_P2_C2_WIP/Powertrain/Electrical Storage System/ ESS Model/Plant/Electrical Plant Model/OCV Estimation/Discharge ==
  SOC [%] : Inport
  1-D Lookup Table1 : Lookup_n-D  NumberOfTableDimensions=1  BreakpointsForDimension1=Plants.ESS.Mdl.Plant.EPM.OCV_Est.SOC  Table=Plants.ESS.Mdl.Plant.EPM.OCV_Est.OCV_Discharge  InternalRulePriority=Speed  RndMeth=Simplest  InputSameDT=on
  OCV [V] : Outport
  wires:
  SOC [%]/1 -> 1-D Lookup Table1/1
  1-D Lookup Table1/1 -> OCV [V]/1

== system EcoSIM3_P2_C2_WIP/Powertrain/Electrical Storage System/ ESS Model/Plant/Electrical Plant Model/Resistance Estimation (Per Cell) /Charge ==
  Temp [C] : Inport
  SOC [%] : Inport  Port=2
  R_1_d1 : Lookup2D  RowIndex=Plants.ESS.Mdl.Plant.EPM.R_Est.Resis_temp_data  ColumnIndex=Plants.ESS.Mdl.Plant.EPM.R_Est.Resis_soc_data  Table=Plants.ESS.Mdl.Plant.EPM.R_Est.Resis_charge_data  LookUpMeth=Interpolation-Use End Values
  R_cell [Ohms] : Outport
  wires:
  Temp [C]/1 -> R_1_d1/1
  SOC [%]/1 -> R_1_d1/2
  R_1_d1/1 -> R_cell [Ohms]/1

== system EcoSIM3_P2_C2_WIP/Powertrain/Electrical Storage System/ ESS Model/Plant/Electrical Plant Model/Resistance Estimation (Per Cell) /Discharge ==
  Temp [C] : Inport
  SOC [%] : Inport  Port=2
  R_1_d1 : Lookup2D  RowIndex=Plants.ESS.Mdl.Plant.EPM.R_Est.Resis_temp_data  ColumnIndex=Plants.ESS.Mdl.Plant.EPM.R_Est.Resis_soc_data  Table=Plants.ESS.Mdl.Plant.EPM.R_Est.Resis_discharge_data  LookUpMeth=Interpolation-Use End Values
  R_cell [Ohms] : Outport
  wires:
  Temp [C]/1 -> R_1_d1/1
  SOC [%]/1 -> R_1_d1/2
  R_1_d1/1 -> R_cell [Ohms]/1

== system EcoSIM3_P2_C2_WIP/Powertrain/Electrical Storage System/Soft ECU/Algorithm/Current Buffer/Charge Buffer/Moderator-Opposer ==
  note: Optimized Gains for buffer depletion:
      | For I*t
      | For I<50 amps
      | Moderator = 0.1247
      | Opposer = 0.4002
      | For I> 50 amps
      | Moderator = 0.0449
      | Opposer = 0.4651
      | For I>50 amps and saturated to 50 amps
      | Moderator = 0.061
      | Opposer = 0.2799
  Current : Inport
  Add2 : Sum  Inputs=+-
  Add5 : Sum  Inputs=+-
  Add6 : Sum  Inputs=+-
  Constant : Constant  Value=100
  Integrator3 : Integrator  LimitOutput=on  UpperSaturationLimit=100
  Moderator : Subsystem
  Opposer : Subsystem
  Saturation2 : Saturate  UpperLimit=100  LowerLimit=0
  Saturation6 : Saturate  UpperLimit=50  LowerLimit=0
  Scope3 : Scope
      settings: SaveName=ScopeData3
  Buffer : Outport
  wires:
  Saturation6/1 -> Add5/1
  Current/1 -> Saturation6/1
  Saturation2/1 -> Buffer/1, Add6/2, Scope3/1
  Add2/1 -> Saturation2/1
  Integrator3/1 -> Add2/2
  Constant/1 -> Add6/1, Add2/1
  Moderator/1(O) -> Integrator3/1
  Add6/1 -> Opposer/1(I)
  Add5/1 -> Moderator/1(I)
  Opposer/1(O) -> Add5/2

== system EcoSIM3_P2_C2_WIP/Powertrain/Electrical Storage System/Soft ECU/Algorithm/Current Buffer/Charge Buffer/RollingAverage ==
  note: 20
  Batt_Current : Inport
  Add3 : Sum  Inputs=+-
  Constant4 : Constant  Value=40
  Gain1 : Gain  Gain=1/0.4
  Saturation1 : Saturate  UpperLimit=100  LowerLimit=0
  Transfer Fcn : TransferFcn  Denominator=[Plants.ESS.SoftECU.Buffer.Charge.TimeConst 1]
  Buffer : Outport
  wires:
  Constant4/1 -> Add3/1
  Gain1/1 -> Saturation1/1
  Saturation1/1 -> Buffer/1
  Add3/1 -> Gain1/1
  Batt_Current/1 -> Transfer Fcn/1
  Transfer Fcn/1 -> Add3/2

== system EcoSIM3_P2_C2_WIP/Powertrain/Electrical Storage System/Soft ECU/Algorithm/Current Buffer/Discharge Buffer/Moderator-Opposer ==
  note: For buffer tor ise back at zero current:
      | Moderator = 0.0413
      | Opposer  = 1.2456
  note: From AcclnTest250
      | For I*t
      | Moderator = 0.0205
      | Opposer = 0.9207
      | For I<130 amps
      | Moderator = 0.0407
      | Opposer = 1.0057
      |
      | For buffer tor ise back at zero current:
      | Moderator = 0.0413
      | Opposer  = 1.2456
  Current : Inport
  Add{1..2,5..6} (4 alike) : Sum  Inputs=+-
  Constant : Constant  Value=100
  Constant3 : Constant  Value=100
  Initial_Disbuf : Constant  Value=100
  Integrator3 : Integrator  InitialConditionSource=external  InitialCondition=11  LimitOutput=on  UpperSaturationLimit=100
  Moderator : Subsystem
  Opposer : Subsystem
  Saturation : Saturate  UpperLimit=130  LowerLimit=0
  Saturation2 : Saturate  UpperLimit=100  LowerLimit=0
  Scope3 : Scope
      settings: SaveName=ScopeData3
  Scope4 : Scope
      settings: SaveName=ScopeData4
  Buffer : Outport
  wires:
  Add6/1 -> Opposer/1(I)
  Constant3/1 -> Add1/1
  Moderator/1(O) -> Integrator3/1
  Integrator3/1 -> Add2/2
  Initial_Disbuf/1 -> Add1/2
  Constant/1 -> Add6/1, Add2/1
  Opposer/1(O) -> Add5/2
  Add1/1 -> Integrator3/2
  Add2/1 -> Scope4/1, Saturation2/1
  Add5/1 -> Moderator/1(I)
  Saturation2/1 -> Buffer/1, Add6/2, Scope3/1
  Saturation/1 -> Add5/1
  Current/1 -> Saturation/1

== system EcoSIM3_P2_C2_WIP/Powertrain/Electrical Storage System/Soft ECU/Algorithm/Current Buffer/Discharge Buffer/RollingAverage ==
  note: 28.725
  Batt_Current : Inport
  Add3 : Sum  Inputs=+-
  Constant4 : Constant  Value=120
  Gain1 : Gain  Gain=1/1.2
  Saturation1 : Saturate  UpperLimit=100  LowerLimit=0
  Transfer Fcn : TransferFcn  Denominator=[Plants.ESS.SoftECU.Buffer.Discharge.TimeConst 1]
  Buffer : Outport
  wires:
  Constant4/1 -> Add3/1
  Gain1/1 -> Saturation1/1
  Saturation1/1 -> Buffer/1
  Add3/1 -> Gain1/1
  Batt_Current/1 -> Transfer Fcn/1
  Transfer Fcn/1 -> Add3/2

== system EcoSIM3_P2_C2_WIP/Powertrain/Engine/Soft ECU/Algorithm/TorqueRegulation/Enabled Subsystem/Delay ==
  Engine_Speed_Rad_per_sec : Inport
  Memory : Memory
  Transfer Fcn1 : TransferFcn  Denominator=[1 1]
  Transport Delay : TransportDelay  Commented=on  DelayTime=0
  Pre_Engine_Speed_Rad_per_sec : Outport
  wires:
  Engine_Speed_Rad_per_sec/1 -> Memory/1
  Memory/1 -> Pre_Engine_Speed_Rad_per_sec/1

== system EcoSIM3_P2_C2_WIP/Powertrain/Engine/Soft ECU/Algorithm/TorqueRegulation/Enabled Subsystem1/Delay ==
  Engine_Speed_Rad_per_sec : Inport
  Memory : Memory
  Transfer Fcn1 : TransferFcn  Denominator=[1 1]
  Transport Delay : TransportDelay  Commented=on  DelayTime=0
  Pre_Engine_Speed_Rad_per_sec : Outport
  wires:
  Memory/1 -> Pre_Engine_Speed_Rad_per_sec/1
  Engine_Speed_Rad_per_sec/1 -> Memory/1

== system EcoSIM3_P2_C2_WIP/Supervisory Controller/Functional Safety1/Functional Safety Algorithm/Fault Detection (Team Developed)/Torque Security Faults/Torque Comparisons/BAS Torque Comparison ==
  In1 : Inport
  Out1 : Outport

== system EcoSIM3_P2_C2_WIP/Supervisory Controller/Functional Safety1/Functional Safety Algorithm/Fault Detection (Team Developed)/Torque Security Faults/Torque Comparisons/Belt Coupler Torque Comparison ==
  In1 : Inport
  Out1 : Outport

== system EcoSIM3_P2_C2_WIP/Supervisory Controller/Functional Safety1/Functional Safety Algorithm/Fault Detection (Team Developed)/Torque Security Faults/Torque Comparisons/Clutch Torque Comparison ==
  In1 : Inport
  Out1 : Outport

== system EcoSIM3_P2_C2_WIP/Supervisory Controller/Functional Safety1/Functional Safety Algorithm/Fault Detection (Team Developed)/Torque Security Faults/Torque Comparisons/Electric Motor Torque Comparison ==
  note: second signal should be torque command from HSC
  In1 : Inport
  Bus Selector : BusSelector  OutputSignals=CAN_Inputs (signal 2).EM_Transmit.EM_Torque_Out_Nm,CAN_Inputs (signal 2).EM_Transmit.EM_Torque_Out_Nm,Torque_Estimates (signal 1).EM_Trq_out_Est_Nm
  Faul_Detect : Subsystem
  Logical Operator2 : Logic  Operator=OR  Inputs=3  AllPortsSameDT=off  OutDataTypeStr=boolean
  Subsystem : Subsystem  Commented=on
  Subsystem1 : Subsystem  Commented=on
  Out1 : Outport
  wires:
  Faul_Detect/1(Fault) -> Logical Operator2/3
  Bus Selector/1 -> Subsystem1/1(Trq Feedback), Faul_Detect/2(Trq feedback)  "<EM_Torque_Out_Nm>"
  Bus Selector/2 -> Subsystem1/2(Trq Req), Subsystem/1(Trq Req)  "<EM_Torque_Out_Nm>"
  Bus Selector/3 -> Subsystem/2(Trq Est), Faul_Detect/1(Trq Est)  "<EM_Trq_out_Est_Nm>"
  Subsystem1/1(Fault) -> Logical Operator2/1
  Subsystem/1(Fault) -> Logical Operator2/2
  Logical Operator2/1 -> Out1/1  "EM_Trq_Fault"
  In1/1 -> Bus Selector/1

== system EcoSIM3_P2_C2_WIP/Supervisory Controller/Functional Safety1/Functional Safety Algorithm/Fault Detection (Team Developed)/Torque Security Faults/Torque Comparisons/Engine Torque Comparison ==
  In1 : Inport
  Out1 : Outport

== system EcoSIM3_P2_C2_WIP/Supervisory Controller/Functional Safety1/Functional Safety Algorithm/Fault Detection (Team Developed)/Torque Security Faults/Torque Comparisons/PTU Torque Comparison ==
  In1 : Inport
  Out1 : Outport

== system EcoSIM3_P2_C2_WIP/Supervisory Controller/Functional Safety1/Functional Safety Algorithm/Fault Detection (Team Developed)/Torque Security Faults/Torque Comparisons/Rear Diff Torque Comparison ==
  In1 : Inport
  Out1 : Outport

== system EcoSIM3_P2_C2_WIP/Supervisory Controller/Functional Safety1/Functional Safety Algorithm/Fault Detection (Team Developed)/Torque Security Faults/Torque Comparisons/Trans Torque Comparison ==
  In1 : Inport
  Out1 : Outport

== system EcoSIM3_P2_C2_WIP/Supervisory Controller/Functional Safety1/Functional Safety Algorithm/Fault Detection (Team Developed)/Torque Security Faults/Torque Comparisons/Wheel Torque Comparison ==
  In1 : Inport
  Ground : Ground
  Terminator : Terminator
  Out1 : Outport
  wires:
  Ground/1 -> Out1/1
  In1/1 -> Terminator/1

== system EcoSIM3_P2_C2_WIP/Supervisory Controller/Functional Safety1/Functional Safety Algorithm/Fault Detection (Team Developed)/Torque Security Faults/Torque Estimation/BAS Torque Estimation ==
  In1 : Inport
  Out1 : Outport

== system EcoSIM3_P2_C2_WIP/Supervisory Controller/Functional Safety1/Functional Safety Algorithm/Fault Detection (Team Developed)/Torque Security Faults/Torque Estimation/Belt Coupler Torque Estimation ==
  In1 : Inport
  Out1 : Outport

== system EcoSIM3_P2_C2_WIP/Supervisory Controller/Functional Safety1/Functional Safety Algorithm/Fault Detection (Team Developed)/Torque Security Faults/Torque Estimation/Clutch Torque Estimation ==
  In1 : Inport
  Out1 : Outport
